simulink model "VelocityControl"  (R2020a)
settings: Solver=VariableStepAuto  StartTime=0.0  StopTime=60  RelTol=2.8421709430404007E-14
values from neighbouring files (symbols this model uses):
  dt_delay = 0.01    [main.m]
  Kd = diag([Kd1; Kd2; Kd3])    [main.m]
  Kd1 = 1/bode(G1, w_crossover)    [main.m]
  Kd2 = 1/bode(G2, w_crossover)    [main.m]
  Kd3 = 1/bode(G3, w_crossover)    [main.m]
  q0_BI = e2q(e, 45*pi/180)    [main.m]
  wbi0_B = [5; -10; 15]*pi/180    [main.m]
  wbi0_P = A_PB*wbi0_B    [main.m]
  wbistar_B = [1;1;1]    [main.m]
undefined symbols (not defined in the file or in its folder): A_BP, A_PB, J_C_B, J_C_P
libraries: simulink_extras x3
settings Model: Creator=bbingham  LastModifiedBy=tjones
settings DataIOCC: SaveOutput=off  SignalLogging=off  DSMLogging=off  ReturnWorkspaceOutputs=off
settings DebuggingCC: ArithmeticOperatorsInVariantConditions=warning
settings SFSimCC: SimUseLocalCustomCode=off  CustomCodeUndefinedFunction=UseInterfaceOnly
settings RTWCC: Description=Simulink Desktop Real-Time  SystemTargetFile=sldrt.tlc  TemplateMakefile=sldrt.tmf  RTWUseLocalCustomCode=off  RTWCompilerOptimization=on
settings CodeAppCC: MaxIdLength=95  StateflowObjectComments=on
settings TargetCC: TargetPreCompLibLocation=C:\Program Files\MATLAB\R2020a\toolbox\sldrt\lib\win64  TargetLangStandard=C99 (ISO)  SupportVariableSizeSignals=on
settings SimscapeCC: SimscapeNormalizeSystem=off

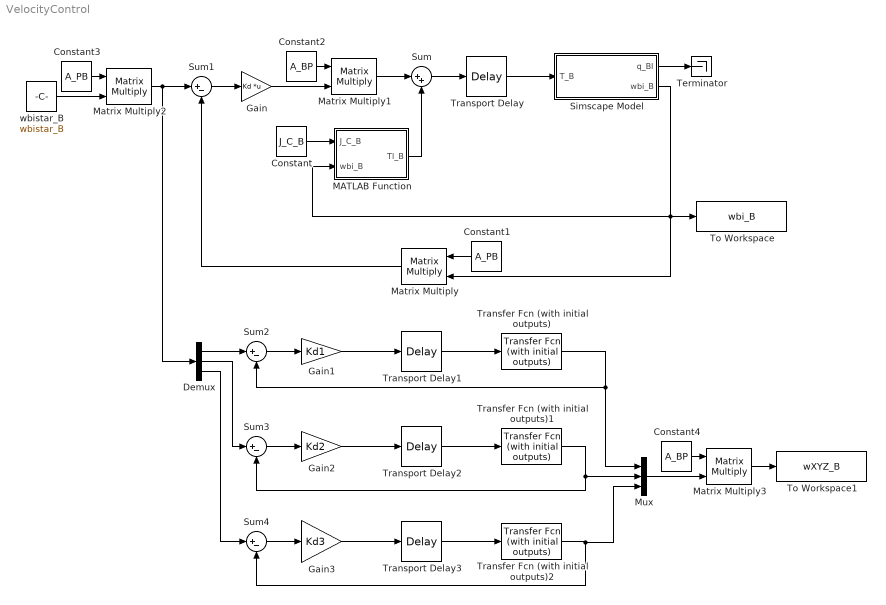
== system VelocityControl ==
  Constant : Constant  Value=J_C_B
  Constant1 : Constant  Value=A_PB
  Constant2 : Constant  Value=A_BP
  Constant3 : Constant  Value=A_PB
  Constant4 : Constant  Value=A_BP
  Demux : Demux  Outputs=3
  Gain : Gain  Gain=Kd  Multiplication=Matrix(K*u) (u vector)
  Gain1 : Gain  Gain=Kd1
  Gain2 : Gain  Gain=Kd2
  Gain3 : Gain  Gain=Kd3
  MATLAB Function : MATLAB Function  TreatAsAtomicUnit=on
  Matrix Multiply{,1..3} (4 alike) : Product  Multiplication=Matrix(*)
  Mux : Mux  Inputs=3
  Simscape Model : Subsystem  TreatAsAtomicUnit=on
  Sum : Sum  Inputs=|++
  Sum{1..4} (4 alike) : Sum  Inputs=|+-
  Terminator : Terminator
  To Workspace : ToWorkspace  VariableName=wbi_B  SaveFormat=Timeseries  SampleTime=-1
  To Workspace1 : ToWorkspace  VariableName=wXYZ_B  SaveFormat=Timeseries  SampleTime=-1
  Transfer Fcn (with initial outputs) : simulink_extras/Additional Linear/Transfer Fcn (with initial outputs)  N=[1]  D="[J_C_P(1,1)  0]"  Y0=wbi0_P(1)  U0=0
  Transfer Fcn (with initial outputs)1 : simulink_extras/Additional Linear/Transfer Fcn (with initial outputs)  N=[1]  D="[J_C_P(2,2)  0]"  Y0=wbi0_P(2)  U0=0
  Transfer Fcn (with initial outputs)2 : simulink_extras/Additional Linear/Transfer Fcn (with initial outputs)  N=[1]  D="[J_C_P(3,3)  0]"  Y0=wbi0_P(3)  U0=0
  Transport Delay{,1..3} (4 alike) : TransportDelay  DelayTime=dt_delay  BufferSize=2048
  wbistar_B : Constant  Value=wbistar_B
  wires:
  Transport Delay/1 -> Simscape Model/1(T_B)
  Simscape Model/1(q_BI) -> Terminator/1
  Sum/1 -> Transport Delay/1
  Simscape Model/2(wbi_B) -> MATLAB Function/2(wbi_B), Matrix Multiply/2, To Workspace/1
  MATLAB Function/1(Tl_B) -> Sum/2
  Constant/1 -> MATLAB Function/1(J_C_B)
  Constant1/1 -> Matrix Multiply/1
  Matrix Multiply/1 -> Sum1/2
  Sum1/1 -> Gain/1
  Constant2/1 -> Matrix Multiply1/1
  Gain/1 -> Matrix Multiply1/2
  Matrix Multiply1/1 -> Sum/1
  Constant3/1 -> Matrix Multiply2/1
  Matrix Multiply2/1 -> Demux/1, Sum1/1
  wbistar_B/1 -> Matrix Multiply2/2
  Gain1/1 -> Transport Delay1/1
  Transport Delay1/1 -> Transfer Fcn (with initial outputs)/1
  Transfer Fcn (with initial outputs)/1 -> Mux/1, Sum2/2
  Sum2/1 -> Gain1/1
  Demux/1 -> Sum2/1
  Sum3/1 -> Gain2/1
  Gain2/1 -> Transport Delay2/1
  Transport Delay2/1 -> Transfer Fcn (with initial outputs)1/1
  Transfer Fcn (with initial outputs)1/1 -> Sum3/2, Mux/2
  Sum4/1 -> Gain3/1
  Gain3/1 -> Transport Delay3/1
  Demux/3 -> Sum4/1
  Transport Delay3/1 -> Transfer Fcn (with initial outputs)2/1
  Transfer Fcn (with initial outputs)2/1 -> Mux/3, Sum4/2
  Demux/2 -> Sum3/1
  Constant4/1 -> Matrix Multiply3/1
  Mux/1 -> Matrix Multiply3/2
  Matrix Multiply3/1 -> To Workspace1/1

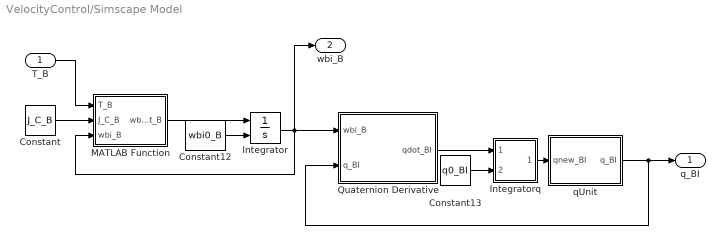
== system VelocityControl/Simscape Model ==
  T_B : Inport
  Constant : Constant  Value=J_C_B
  Constant12 : Constant  Value=wbi0_B
  Constant13 : Constant  Value=q0_BI  OutDataTypeStr=Bus: qBus
  Integrator : Integrator  InitialConditionSource=external
  Integratorq : Subsystem
  MATLAB Function : MATLAB Function  TreatAsAtomicUnit=on
  Quaternion Derivative : MATLAB Function  TreatAsAtomicUnit=on
  qUnit : MATLAB Function  TreatAsAtomicUnit=on
  q_BI : Outport  OutDataTypeStr=Bus: qBus  VectorParamsAs1DForOutWhenUnconnected=off
  wbi_B : Outport  Port=2  VectorParamsAs1DForOutWhenUnconnected=off
  wires:
  qUnit/1(q_BI) -> q_BI/1, Quaternion Derivative/2(q_BI)
  Integratorq/1(qnew_BI) -> qUnit/1(qnew_BI)
  Quaternion Derivative/1(qdot_BI) -> Integratorq/1(qdot_BI)
  Constant13/1 -> Integratorq/2(q0_BI)
  MATLAB Function/1(wbidot_B) -> Integrator/1
  Constant12/1 -> Integrator/2
  Constant/1 -> MATLAB Function/2(J_C_B)
  Integrator/1 -> wbi_B/1, MATLAB Function/3(wbi_B), Quaternion Derivative/1(wbi_B)
  T_B/1 -> MATLAB Function/1(T_B)

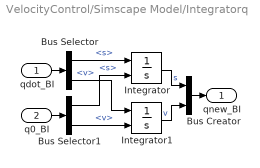
== system VelocityControl/Simscape Model/Integratorq ==
  qdot_BI : Inport  OutDataTypeStr=Bus: qBus
  q0_BI : Inport  Port=2  OutDataTypeStr=Bus: qBus
  Bus Creator : BusCreator  Inputs=2  OutDataTypeStr=Bus: qBus
      settings: InheritFromInputs=off
  Bus Selector : BusSelector  OutputSignals=s,v
  Bus Selector1 : BusSelector  OutputSignals=s,v
  Integrator : Integrator  InitialConditionSource=external
  Integrator1 : Integrator  InitialConditionSource=external
  qnew_BI : Outport  OutDataTypeStr=Bus: qBus  VectorParamsAs1DForOutWhenUnconnected=off
  wires:
  qdot_BI/1 -> Bus Selector/1
  q0_BI/1 -> Bus Selector1/1
  Bus Selector/1 -> Integrator/1  "<s>"
  Bus Selector1/1 -> Integrator/2  "<s>"
  Bus Selector/2 -> Integrator1/1  "<v>"
  Bus Selector1/2 -> Integrator1/2  "<v>"
  Integrator/1 -> Bus Creator/1  "s"
  Integrator1/1 -> Bus Creator/2  "v"
  Bus Creator/1 -> qnew_BI/1

== matlab function VelocityControl/MATLAB Function ==
  data: J_C_B input; Tl_B output; wbi_B input
function Tl_B = fcn(J_C_B, wbi_B)

Tl_B = cross(wbi_B, J_C_B*wbi_B);

== matlab function VelocityControl/Simscape Model/Quaternion Derivative ==
  data: wbi_B input; q_BI input Bus: qBus; qdot_BI output Bus: qBus
function qdot_BI = fcn(wbi_B, q_BI)

w.s = 0;
w.v = wbi_B;

qdot = qX(w, q_BI);

qdot_BI.s = 1/2*qdot.s;
qdot_BI.v = 1/2*qdot.v;

== matlab function VelocityControl/Simscape Model/qUnit ==
  data: qnew_BI input Bus: qBus; q_BI output Bus: qBus
function q_BI = fcn(qnew_BI)

q_BI = qUnit(qnew_BI);

== matlab function VelocityControl/Simscape Model/MATLAB Function ==
  data: T_B input; wbidot_B output; J_C_B input; wbi_B input
function wbidot_B = fcn(T_B, J_C_B, wbi_B)

wbidot_B = J_C_B\(T_B - cross(wbi_B, J_C_B*wbi_B));
